simulink model "PI_Controlled_SAPF_pq_theory"  (R2023b)
settings: Solver=VariableStepAuto  StartTime=0.0  StopTime=10  RelTol=1e-3
undefined symbols (not defined in the file): DiscIntNeverNeededParam
libraries: spsThreePhaseVIMeasurementLib x3, spsSeriesRLCBranchLib x2, spsUniversalBridgeLib x2, dspfdesign x1, spsThreePhaseSeriesRLCBranchLib x1, spsThreePhaseSourceLib x1, spsVoltageMeasurementLib x1, spspowerguiLib x1
settings Model: Creator=Nitiz Khanal  LastModifiedBy=khana
settings DataIOCC: ReturnWorkspaceOutputs=off

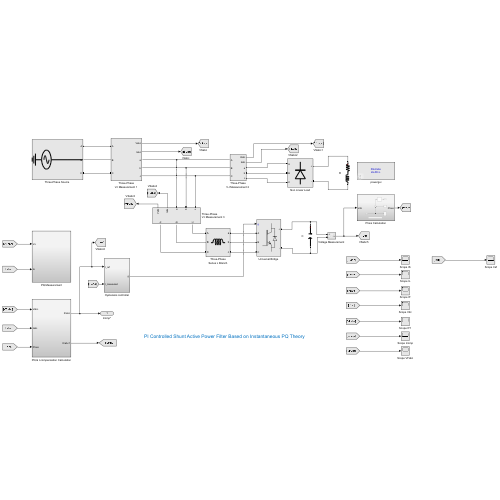
[thumbnail: Simulink's stored preview of the top-level diagram]
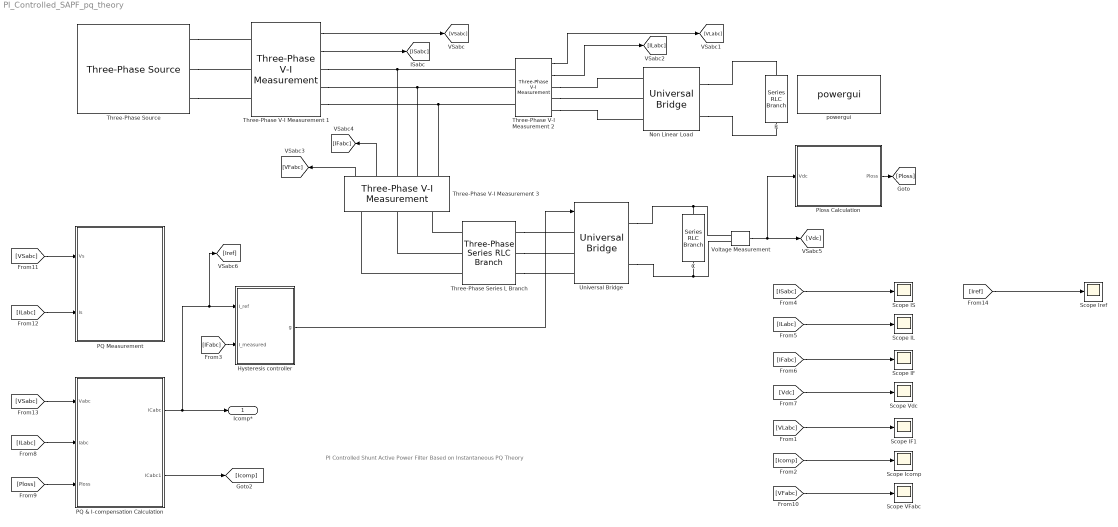
== system PI_Controlled_SAPF_pq_theory ==
  note: PI Controlled Shunt Active Power Filter Based on Instantaneous PQ Theory
  C : spsSeriesRLCBranchLib/Series RLC Branch  LConnTagsString=__new0  RConnTagsString=__new0  BranchType=C  Resistance=1  Inductance=1e-3  SetiL0=off  InitialCurrent=0  Capacitance=1500e-6  Setx0=on  InitialVoltage=500  Measurements=None
  Hysteresis controller : Subsystem
  Non Linear Load : spsUniversalBridgeLib/Universal Bridge  Arms=3  SnubberResistance=1e5  SnubberCapacitance=inf  Device=Diodes  Ron=1e-3  Lon=0  ForwardVoltages="[  0  0  ]"  ForwardVoltage=0  GTOparameters=[ 10e-6 , 20e-6 ]  IGBTparameters=[ 1e-6 , 2e-6 ]  Measurements=None  Measurements_2=None  converterType=Rectifier
  PQ & I-compensation Calculation : Subsystem
  PQ Measurement : Subsystem
  Ploss Calculation : Subsystem
  R : spsSeriesRLCBranchLib/Series RLC Branch  LConnTagsString=__new0  RConnTagsString=__new0  BranchType=RL  Resistance=30  Inductance=100e-3  SetiL0=off  InitialCurrent=0  Capacitance=1e-6  Setx0=off  InitialVoltage=0  Measurements=None
  Scope IF : Scope
  Scope IF1 : Scope
  Scope IL : Scope
  Scope IS : Scope
  Scope Icomp : Scope
  Scope Iref : Scope
  Scope VFabc : Scope
  Scope Vdc : Scope
  Three-Phase Series L Branch : spsThreePhaseSeriesRLCBranchLib/Three-Phase Series RLC Branch  LConnTagsString=A|B|C  RConnTagsString=A|B|C  BranchType=L  Resistance=1  Inductance=2e-3  Capacitance=1e-6  Measurements=None
  "Three-Phase V-I Measurement 1 " : spsThreePhaseVIMeasurementLib/Three-Phase V-I Measurement  VoltageMeasurement=phase-to-ground  SetLabelV=off  LabelV=Vabc  Vpu=off  VpuLL=off  CurrentMeasurement=yes  SetLabelI=off  LabelI=Iabc  Ipu=off  Pbase=100e6  Vbase=500e3  OutputType=Complex  PhasorSimulation=off  PSBequivalent=0
  "Three-Phase V-I Measurement 2 " : spsThreePhaseVIMeasurementLib/Three-Phase V-I Measurement  VoltageMeasurement=phase-to-ground  SetLabelV=off  LabelV=Vabc  Vpu=off  VpuLL=off  CurrentMeasurement=yes  SetLabelI=off  LabelI=Iabc  Ipu=off  Pbase=100e6  Vbase=500e3  OutputType=Complex  PhasorSimulation=off  PSBequivalent=0
  Three-Phase V-I Measurement 3 : spsThreePhaseVIMeasurementLib/Three-Phase V-I Measurement  VoltageMeasurement=phase-to-ground  SetLabelV=off  LabelV=Vabc  Vpu=off  VpuLL=off  CurrentMeasurement=yes  SetLabelI=off  LabelI=Iabc  Ipu=off  Pbase=100e6  Vbase=500e3  OutputType=Complex  PhasorSimulation=off  PSBequivalent=0
  "Three-Phase Source " : spsThreePhaseSourceLib/Three-Phase Source  InternalConnection=Yg  VoltagePhases=off  Voltage=220  PhaseAngle=0  Voltage_phases=[25e3 25e3 25e3]/sqrt(3)  PhaseAngles_phases=[0 -120 +120]  Frequency=50  NonIdealSource=off  SpecifyImpedance=off  Resistance=0.8929  Inductance=16.58e-3  ShortCircuitLevel=100e6  BaseVoltage=25e3  XRratio=7  BusType=swing  Pref=10e3  Qref=0  Prefabc=[10e3, 10e3, 10e3]  Qrefabc=[0, 0, 0]  Qmin=-inf  Qmax=inf
  "Universal Bridge " : spsUniversalBridgeLib/Universal Bridge  Arms=3  SnubberResistance=1e5  SnubberCapacitance=inf  Device=IGBT / Diodes  Ron=1e-3  Lon=0  ForwardVoltages="[  0  0  ]"  ForwardVoltage=0  GTOparameters=[ 10e-6 , 20e-6 ]  IGBTparameters=[ 1e-6 , 2e-6 ]  Measurements=None  Measurements_2=None  converterType=Rectifier
  "Voltage Measurement " : spsVoltageMeasurementLib/Voltage Measurement  PhasorSimulation=off  OutputType=Complex  PSBequivalent=0
  powergui : spspowerguiLib/powergui  Priority=1  SimulationMode=Discrete  SampleTime=2e-6  frequency=60  Iterations=50  frequencyindice=50  Pbase=100e6  ErrMax=1e-4  UnitsV=kV  UnitsW=MW  buscounter=0  FunctionMessages=off  echomessages=off  EnableUseOfTLC=off  CurrentSourceSwitches=off  DisableSnubberDevices=off  DisableRonSwitches=off  DisableVfSwitches=off  DisplayEquations=off  AutomaticDiscreteSolvers=off  SolverType=Tustin/Backward Euler (TBE)  Interpol=off  ExternalGateDelay=off  methode=off  Ts=100  x0status=blocks  SPID=on  SwTol=0  HookPort=off  NonlinearTolerance=1e-4  nMaxIteration=100  ContinueOnMaxIteration=off  RestoreLinks=warning  ResistiveCurrentMeasurement=off  Frange=[0:2:500]  Ylog=off  Xlog=on  ShowGrid=off  save=off  variable=ZData  structure=0  ZoomFFT=off  StartTime=0.0  cycles=1  DisplayStyle=1  fundamental=60  FreqAxis=off  MaxFrequency=1000  frequencyindicesteady=1  RmsSteady=1  display=off
  Icomp* : Outport
  wires:
  "Three-Phase V-I Measurement 1 "/1 -> [VSabc]
  "Three-Phase V-I Measurement 1 "/2 -> [ISabc]
  "Three-Phase V-I Measurement 2 "/1 -> [VLabc]
  "Three-Phase V-I Measurement 2 "/2 -> [ILabc]
  Three-Phase V-I Measurement 3/1 -> [VFabc]
  Three-Phase V-I Measurement 3/2 -> [IFabc]
  "Voltage Measurement "/1 -> Ploss Calculation/1(Vdc), [Vdc]
  Hysteresis controller/1(g) -> "Universal Bridge "/1
  [ISabc] -> Scope IS/1
  [ILabc] -> Scope IL/1
  [IFabc] -> Scope IF/1
  [Vdc] -> Scope Vdc/1
  Ploss Calculation/1(Ploss) -> [Ploss]
  [VSabc] -> PQ Measurement/1(Vs)
  [ILabc] -> PQ Measurement/2(Is)
  [VSabc] -> PQ & I-compensation Calculation/1(Vabc)
  [IFabc] -> Hysteresis controller/2(I_measured)
  [ILabc] -> PQ & I-compensation Calculation/2(Iabc)
  [Ploss] -> PQ & I-compensation Calculation/3(Ploss)
  PQ & I-compensation Calculation/1(ICabc) -> [Iref], Hysteresis controller/1(I_ref), Icomp*/1
  PQ & I-compensation Calculation/2(ICabc1) -> [Icomp]
  [VLabc] -> Scope IF1/1
  [Icomp] -> Scope Icomp/1
  [VFabc] -> Scope VFabc/1
  [Iref] -> Scope Iref/1
  connections:
  "Three-Phase Source "/RConn1 -- "Three-Phase V-I Measurement 1 "/LConn1
  "Three-Phase Source "/RConn2 -- "Three-Phase V-I Measurement 1 "/LConn2
  "Three-Phase Source "/RConn3 -- "Three-Phase V-I Measurement 1 "/LConn3
  "Three-Phase V-I Measurement 1 "/RConn1 -- Three-Phase V-I Measurement 3/RConn1 -- "Three-Phase V-I Measurement 2 "/LConn1
  "Three-Phase V-I Measurement 1 "/RConn2 -- Three-Phase V-I Measurement 3/RConn2 -- "Three-Phase V-I Measurement 2 "/LConn2
  "Three-Phase V-I Measurement 1 "/RConn3 -- Three-Phase V-I Measurement 3/RConn3 -- "Three-Phase V-I Measurement 2 "/LConn3
  "Three-Phase V-I Measurement 2 "/RConn1 -- Non Linear Load/LConn1
  "Three-Phase V-I Measurement 2 "/RConn2 -- Non Linear Load/LConn2
  "Three-Phase V-I Measurement 2 "/RConn3 -- Non Linear Load/LConn3
  Non Linear Load/RConn1 -- R/LConn1
  Non Linear Load/RConn2 -- R/RConn1
  Three-Phase Series L Branch/RConn1 -- "Universal Bridge "/LConn1
  Three-Phase Series L Branch/RConn2 -- "Universal Bridge "/LConn2
  Three-Phase Series L Branch/RConn3 -- "Universal Bridge "/LConn3
  Three-Phase Series L Branch/LConn1 -- Three-Phase V-I Measurement 3/LConn3
  Three-Phase Series L Branch/LConn2 -- Three-Phase V-I Measurement 3/LConn2
  Three-Phase Series L Branch/LConn3 -- Three-Phase V-I Measurement 3/LConn1
  "Universal Bridge "/RConn1 -- C/LConn1 -- "Voltage Measurement "/LConn1
  "Universal Bridge "/RConn2 -- C/RConn1 -- "Voltage Measurement "/LConn2

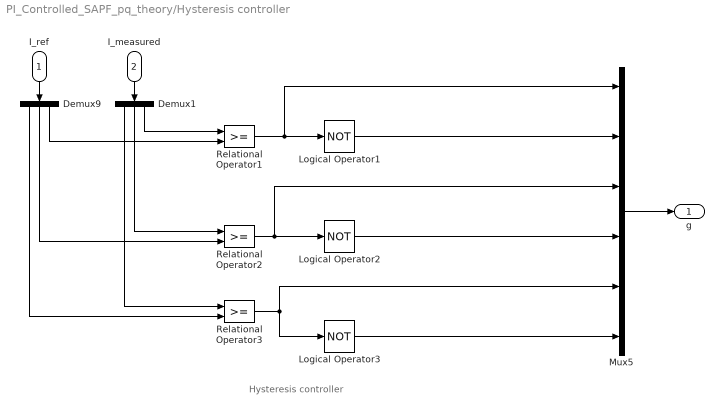
== system PI_Controlled_SAPF_pq_theory/Hysteresis controller ==
  note: Hysteresis controller
  I_ref : Inport
  I_measured : Inport  Port=2
  Demux1 : Demux  Outputs=3
  Demux9 : Demux  Outputs=3
  Logical Operator1 : Logic  Operator=NOT  AllPortsSameDT=off  OutDataTypeStr=boolean
  Logical Operator2 : Logic  Operator=NOT  AllPortsSameDT=off  OutDataTypeStr=boolean
  Logical Operator3 : Logic  Operator=NOT  AllPortsSameDT=off  OutDataTypeStr=boolean
  Mux5 : Mux  Inputs=6
  Relational Operator1 : RelationalOperator  OutDataTypeStr=boolean  InputSameDT=off
  Relational Operator2 : RelationalOperator  OutDataTypeStr=boolean  InputSameDT=off
  Relational Operator3 : RelationalOperator  OutDataTypeStr=boolean  InputSameDT=off
  g : Outport
  wires:
  Relational Operator1/1 -> Logical Operator1/1, Mux5/1
  Relational Operator2/1 -> Logical Operator2/1, Mux5/3
  Relational Operator3/1 -> Logical Operator3/1, Mux5/5
  Logical Operator1/1 -> Mux5/2
  Logical Operator2/1 -> Mux5/4
  Logical Operator3/1 -> Mux5/6
  Mux5/1 -> g/1
  I_ref/1 -> Demux9/1
  I_measured/1 -> Demux1/1
  Demux1/3 -> Relational Operator1/1
  Demux1/2 -> Relational Operator2/1
  Demux1/1 -> Relational Operator3/1
  Demux9/3 -> Relational Operator1/2
  Demux9/2 -> Relational Operator2/2
  Demux9/1 -> Relational Operator3/2

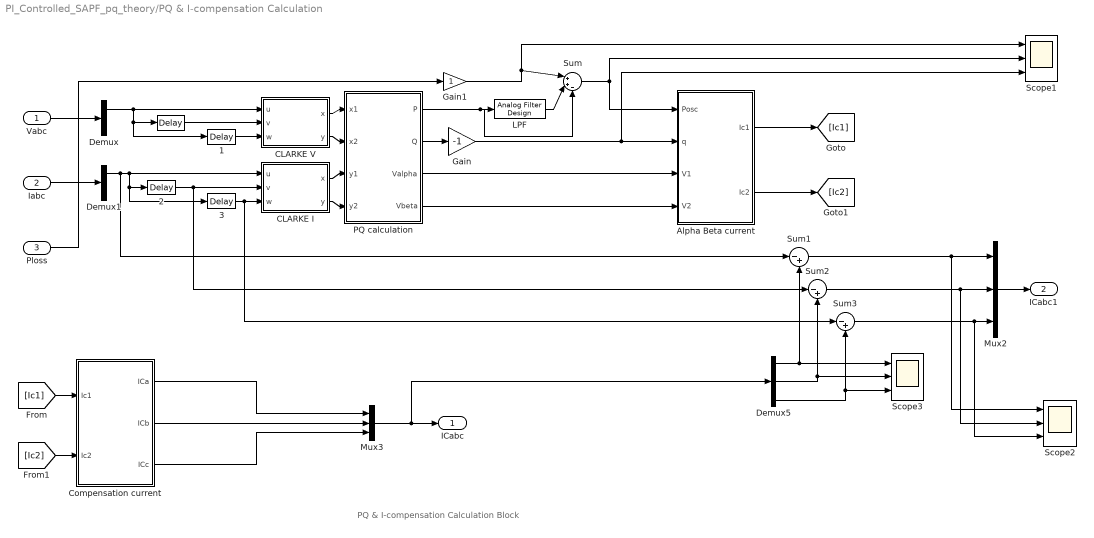
== system PI_Controlled_SAPF_pq_theory/PQ & I-compensation Calculation ==
  note: PQ & I-compensation Calculation Block
  Vabc : Inport
  Iabc : Inport  Port=2
  Ploss : Inport  Port=3
  " " : TransportDelay  DelayTime=0.006666666
  " 1" : TransportDelay  DelayTime=0.013333333
  " 2" : TransportDelay  DelayTime=0.006666666
  " 3" : TransportDelay  DelayTime=0.013333333
  Alpha Beta current : MATLAB Function  TreatAsAtomicUnit=on
  CLARKE I : MATLAB Function  TreatAsAtomicUnit=on
  CLARKE V : MATLAB Function  TreatAsAtomicUnit=on
  Compensation current : MATLAB Function  TreatAsAtomicUnit=on
  Demux : Demux  Outputs=3
  Demux1 : Demux  Outputs=3
  Demux5 : Demux  Outputs=3
  Gain : Gain  Gain=-1
  Gain1 : Gain
  LPF : dspfdesign/Analog Filter Design  method=Butterworth  filttype=Lowpass  N=5  Wlo=2*pi*50  Whi=80  Rp=2  Rs=40
  Mux2 : Mux  Inputs=3
  Mux3 : Mux  Inputs=3
  PQ calculation : MATLAB Function  TreatAsAtomicUnit=on
  Scope1 : Scope  NumInputPorts=3
  Scope2 : Scope  NumInputPorts=3
  Scope3 : Scope  NumInputPorts=3
  Sum : Sum  Inputs=|++-
  Sum1 : Sum  Inputs=|-+
  Sum2 : Sum  Inputs=|-+
  Sum3 : Sum  Inputs=|-+
  ICabc : Outport
  ICabc1 : Outport  Port=2
  wires:
  Iabc/1 -> Demux1/1
  Vabc/1 -> Demux/1
  [Ic1] -> Compensation current/1(Ic1)
  [Ic2] -> Compensation current/2(Ic2)
  Compensation current/1(ICa) -> Mux3/1
  Compensation current/2(ICb) -> Mux3/2
  Compensation current/3(ICc) -> Mux3/3
  CLARKE V/1(x) -> PQ calculation/1(x1)
  CLARKE V/2(y) -> PQ calculation/2(x2)
  CLARKE I/1(x) -> PQ calculation/3(y1)
  PQ calculation/2(Q) -> Gain/1
  PQ calculation/1(P) -> LPF/1, Sum/3
  Gain/1 -> Alpha Beta current/2(q), Scope1/3
  PQ calculation/3(Valpha) -> Alpha Beta current/3(V1)
  Alpha Beta current/1(Ic1) -> [Ic1]
  Alpha Beta current/2(Ic2) -> [Ic2]
  CLARKE I/2(y) -> PQ calculation/4(y2)
  PQ calculation/4(Vbeta) -> Alpha Beta current/4(V2)
  Demux/1 -> CLARKE V/1(u), " "/1, " 1"/1
  Demux1/1 -> CLARKE I/1(u), " 3"/1, " 2"/1, Sum1/1
  LPF/1 -> Sum/2
  Sum/1 -> Alpha Beta current/1(Posc), Scope1/2
  Gain1/1 -> Sum/1, Scope1/1
  Mux3/1 -> ICabc/1, Demux5/1
  Demux5/1 -> Sum1/2, Scope3/1
  Demux5/2 -> Sum2/2, Scope3/2
  Demux5/3 -> Sum3/2, Scope3/3
  Ploss/1 -> Gain1/1
  Sum1/1 -> Mux2/1, Scope2/1
  Sum2/1 -> Mux2/2, Scope2/2
  Sum3/1 -> Mux2/3, Scope2/3
  Mux2/1 -> ICabc1/1
  " "/1 -> CLARKE V/2(v)
  " 1"/1 -> CLARKE V/3(w)
  " 2"/1 -> CLARKE I/2(v), Sum2/1
  " 3"/1 -> CLARKE I/3(w), Sum3/1

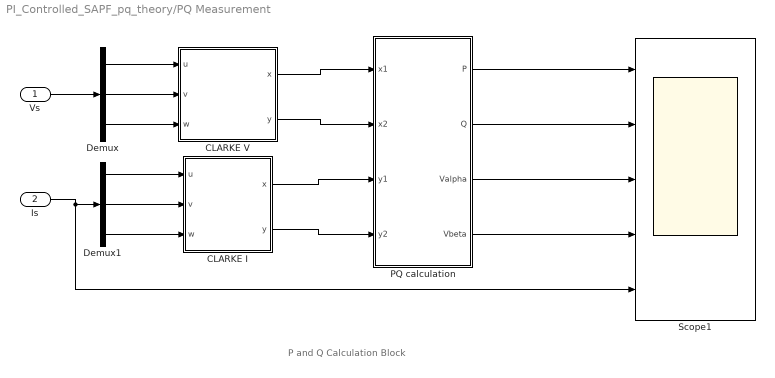
== system PI_Controlled_SAPF_pq_theory/PQ Measurement ==
  note: P and Q Calculation Block
  Vs : Inport
  Is : Inport  Port=2
  CLARKE I : MATLAB Function  TreatAsAtomicUnit=on
  CLARKE V : MATLAB Function  TreatAsAtomicUnit=on
  Demux : Demux  Outputs=3
  Demux1 : Demux  Outputs=3
  PQ calculation : MATLAB Function  TreatAsAtomicUnit=on
  "Scope1 " : Scope  NumInputPorts=5
  wires:
  CLARKE V/1(x) -> PQ calculation/1(x1)
  CLARKE V/2(y) -> PQ calculation/2(x2)
  CLARKE I/1(x) -> PQ calculation/3(y1)
  CLARKE I/2(y) -> PQ calculation/4(y2)
  Demux/1 -> CLARKE V/1(u)
  Demux/2 -> CLARKE V/2(v)
  Demux/3 -> CLARKE V/3(w)
  Demux1/1 -> CLARKE I/1(u)
  Demux1/2 -> CLARKE I/2(v)
  Demux1/3 -> CLARKE I/3(w)
  Vs/1 -> Demux/1
  Is/1 -> Demux1/1, "Scope1 "/5
  PQ calculation/1(P) -> "Scope1 "/1
  PQ calculation/2(Q) -> "Scope1 "/2
  PQ calculation/3(Valpha) -> "Scope1 "/3
  PQ calculation/4(Vbeta) -> "Scope1 "/4

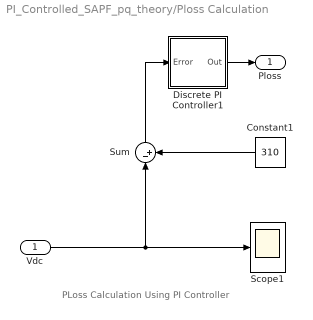
== system PI_Controlled_SAPF_pq_theory/Ploss Calculation ==
  note: PLoss Calculation Using PI Controller
  Vdc : Inport
  Constant1 : Constant  Value=310
  Discrete PI Controller1 : Subsystem  AncestorBlock=|  DialogController=POWERSYS.PowerSysDialog  mask(Discrete PI Controller){Kp=0.1, Ki=0.1, Par_Limits=[1e6 -1e6], Init=0, Ts=5e-6}
      | powerlib_extras/Discrete 
      | Control Blocks/Discrete
      | PI Controller
      mask prompts: Kp "Proportional gain (Kp):"; Ki "Integral gain (Ki):"; Par_Limits "Output limits: [ Upper   Lower ]"; Init "Output initial value:"; Ts "Sample time:"
      mask help: This block implements a discrete PI controller.
      mask init:
      | UpperLimit=Par_Limits(1);
      | LowerLimit=Par_Limits(2);
      | power_initmask();
      settings: LibrarySourceBlock=|
      | powerlib_extras/Discrete
      | Control Blocks/Discrete
      | PI Controller
      mask Help: This block is part of a subset of blocks in the Extras library that does not have documentation associated with it, other than the block mask description.
      mask Display: disp('PI');
  Scope1 : Scope
  Sum : Sum  Inputs=|-+
  Ploss : Outport
  wires:
  Constant1/1 -> Sum/2
  Discrete PI Controller1/1(Out) -> Ploss/1
  Sum/1 -> Discrete PI Controller1/1(Error)
  Vdc/1 -> Sum/1, Scope1/1

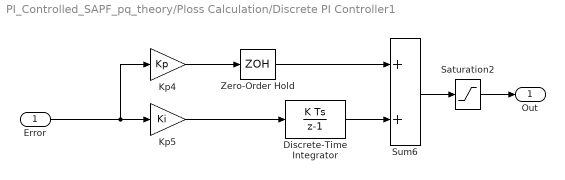
== system PI_Controlled_SAPF_pq_theory/Ploss Calculation/Discrete PI Controller1 ==
  Error : Inport  SampleTime=Ts
  Discrete-Time Integrator : DiscreteIntegrator  InitialCondition=Init  SampleTime=Ts  LimitOutput=on  UpperSaturationLimit=UpperLimit  LowerSaturationLimit=LowerLimit  ICPrevOutput=DiscIntNeverNeededParam  ICPrevScaledInput=DiscIntNeverNeededParam
  Kp4 : Gain  Gain=Kp  SaturateOnIntegerOverflow=on  SampleTime=Ts  OutDataTypeStr=Inherit: Same as input  ParamDataTypeStr=Inherit: Same as input
  Kp5 : Gain  Gain=Ki  SaturateOnIntegerOverflow=on  SampleTime=Ts  OutDataTypeStr=Inherit: Same as input  ParamDataTypeStr=Inherit: Same as input
  Saturation2 : Saturate  UpperLimit=UpperLimit  LowerLimit=LowerLimit  SampleTime=Ts
  Sum6 : Sum  InputSameDT=on  SaturateOnIntegerOverflow=on  SampleTime=Ts  OutDataTypeStr=Inherit: Same as first input
  Zero-Order Hold : ZeroOrderHold  SampleTime=Ts
  Out : Outport  SampleTime=Ts  InitialOutput=0  VectorParamsAs1DForOutWhenUnconnected=off
  wires:
  Zero-Order Hold/1 -> Sum6/1
  Saturation2/1 -> Out/1
  Discrete-Time Integrator/1 -> Sum6/2
  Kp4/1 -> Zero-Order Hold/1
  Kp5/1 -> Discrete-Time Integrator/1
  Sum6/1 -> Saturation2/1
  Error/1 -> Kp5/1, Kp4/1

== matlab function PI_Controlled_SAPF_pq_theory/PQ Measurement/CLARKE I ==
  data: u input; x output; v input; w input; y output
% Clarke Transformation for Current

function [x,y] = ICT(u,v,w)

x = sqrt(2/3)*(u-(0.5*v)-(0.5*w));
y = sqrt(2)*(0+(0.5*v)-(0.5*w));

== matlab function PI_Controlled_SAPF_pq_theory/PQ Measurement/CLARKE V ==
  data: u input; x output; v input; w input; y output
% Clarke Transformation for voltage
function [x,y] = VCT(u,v,w)

x = sqrt(2/3)*(u-(0.5*v)-(0.5*w));
y = sqrt(2)*(0+(0.5*v)-(0.5*w));

== matlab function PI_Controlled_SAPF_pq_theory/PQ Measurement/PQ calculation ==
  data: x1 input; P output; Q output; x2 input; y1 input; y2 input; Valpha output; Vbeta output
%Calculation of P and Q

function [P,Q,Valpha,Vbeta] = PQ(x1,x2,y1,y2)

P = (x1*y1)+(x2*y2);
Q = (x2*y1)-(x1*y2);
Valpha = x1;
Vbeta = x2;

== matlab function PI_Controlled_SAPF_pq_theory/PQ & I-compensation Calculation/Alpha Beta current ==
  data: Posc input; Ic1 output; q input; V1 input; Ic2 output; V2 input
%Calculation of Alpha Beta Calculation

function [Ic1,Ic2] = ICOM(Posc,q,V1,V2)


Ic1 = (-1/(V1^2 + V2^2))*((Posc*V1)+(q*V2));
Ic2 = (-1/(V1^2 + V2^2))*((Posc*V2)-(q*V1));

== matlab function PI_Controlled_SAPF_pq_theory/PQ & I-compensation Calculation/CLARKE I ==
  data: u input; x output; v input; w input; y output
% Clarke Transformation for Current

function [x,y] = ICT(u,v,w)

x = sqrt(2/3)*(u-(0.5*v)-(0.5*w));
y = sqrt(2)*(0+(0.5*v)-(0.5*w));

== matlab function PI_Controlled_SAPF_pq_theory/PQ & I-compensation Calculation/CLARKE V ==
  data: u input; x output; v input; w input; y output
% Clarke Transformation for voltage

function [x,y] = VCT(u,v,w)

x = sqrt(2/3)*(u-(0.5*v)-(0.5*w));
y = sqrt(2)*(0+(0.5*v)-(0.5*w));

== matlab function PI_Controlled_SAPF_pq_theory/PQ & I-compensation Calculation/Compensation current ==
  data: Ic1 input; ICa output; Ic2 input; ICb output; ICc output
%Calculation of Compensating Current
function [ICa,ICb,ICc] = Ical(Ic1,Ic2)

ICa = sqrt(2/3)*(Ic1);
ICb = sqrt(2/3)*((-0.5*Ic1)+((sqrt(3)/2)*Ic2));
ICc = sqrt(2/3)*((-0.5*Ic1)-((sqrt(3)/2)*Ic2));

== matlab function PI_Controlled_SAPF_pq_theory/PQ & I-compensation Calculation/PQ calculation ==
  data: x1 input; P output; Q output; x2 input; y1 input; y2 input; Valpha output; Vbeta output
% P and Q calculation

function [P,Q,Valpha,Vbeta] = PQ(x1,x2,y1,y2)

P = (x1*y1)+(x2*y2);
Q = (x2*y1)-(x1*y2);
Valpha = x1;
Vbeta = x2;
